simulink model "semi_GSTA"  (R2018b)
settings: Solver=FixedStepAuto  StartTime=0.0  StopTime=100  FixedStep=0.01  RelTol=1e-3
InitFcn:
  | parameters_semi_const_noise
model workspace: external: MAT-File (data not in the file)
undefined symbols (not defined in the file or in its folder): eta0, ev_sampling_time, fig_st, h_ATD, h_ATD_sds, Mn, st_controller, T0, v0, x1, x2, x3, x4, x5, x6
libraries: sdolib x6, simulink x1
(part 6 of 6)

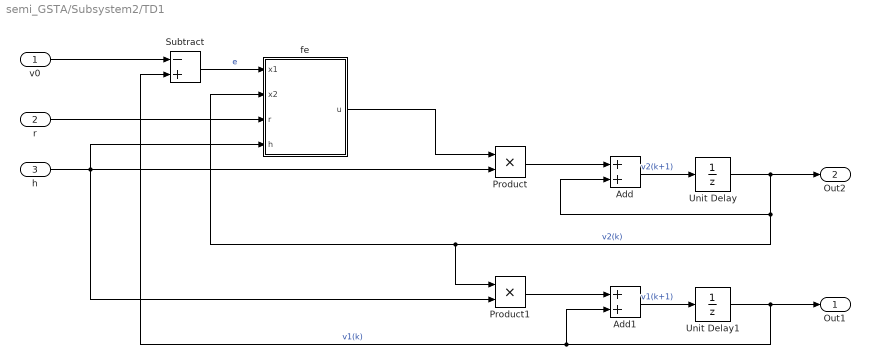
== system semi_GSTA/Subsystem2/TD1 ==
  v0 : Inport
  r : Inport  Port=2
  h : Inport  Port=3
  Add : Sum
  Add1 : Sum
  Product : Product  RndMeth=Zero
  Product1 : Product  RndMeth=Zero
  Subtract : Sum  Inputs=-+
  Unit Delay : UnitDelay  SampleTime=-1
  Unit Delay1 : UnitDelay  InitialCondition=eta0(1)  SampleTime=-1
  fe : MATLAB Function  TreatAsAtomicUnit=on
  Out1 : Outport
  Out2 : Outport  Port=2
  wires:
  v0/1 -> Subtract/1
  Subtract/1 -> fe/1(x1)  "e"
  r/1 -> fe/3(r)
  h/1 -> Product/2, fe/4(h), Product1/2
  fe/1(u) -> Product/1
  Product/1 -> Add/1
  Add/1 -> Unit Delay/1  "v2(k+1)"
  Unit Delay/1 -> Add/2, Product1/1, fe/2(x2), Out2/1  "v2(k)"
  Add1/1 -> Unit Delay1/1  "v1(k+1)"
  Unit Delay1/1 -> Out1/1, Add1/2, Subtract/2  "v1(k)"
  Product1/1 -> Add1/1

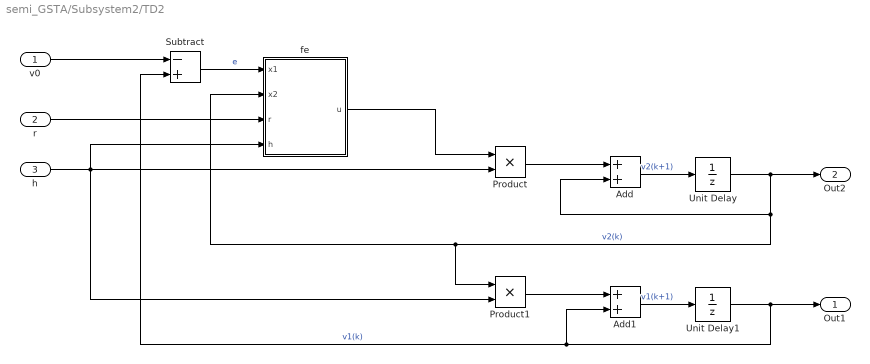
== system semi_GSTA/Subsystem2/TD2 ==
  v0 : Inport
  r : Inport  Port=2
  h : Inport  Port=3
  Add : Sum
  Add1 : Sum
  Product : Product  RndMeth=Zero
  Product1 : Product  RndMeth=Zero
  Subtract : Sum  Inputs=-+
  Unit Delay : UnitDelay  SampleTime=-1
  Unit Delay1 : UnitDelay  InitialCondition=eta0(2)  SampleTime=-1
  fe : MATLAB Function  TreatAsAtomicUnit=on
  Out1 : Outport
  Out2 : Outport  Port=2
  wires:
  Product1/1 -> Add1/1
  Unit Delay1/1 -> Subtract/2, Add1/2, Out1/1  "v1(k)"
  Add1/1 -> Unit Delay1/1  "v1(k+1)"
  Unit Delay/1 -> Out2/1, fe/2(x2), Product1/1, Add/2  "v2(k)"
  Add/1 -> Unit Delay/1  "v2(k+1)"
  Product/1 -> Add/1
  fe/1(u) -> Product/1
  h/1 -> Product1/2, fe/4(h), Product/2
  r/1 -> fe/3(r)
  Subtract/1 -> fe/1(x1)  "e"
  v0/1 -> Subtract/1

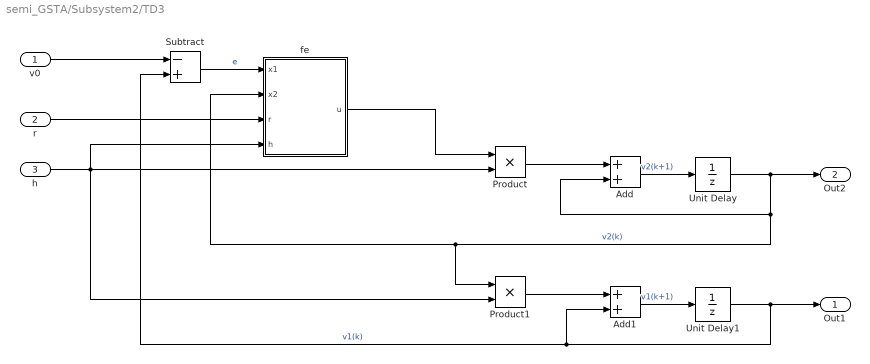
== system semi_GSTA/Subsystem2/TD3 ==
  v0 : Inport
  r : Inport  Port=2
  h : Inport  Port=3
  Add : Sum
  Add1 : Sum
  Product : Product  RndMeth=Zero
  Product1 : Product  RndMeth=Zero
  Subtract : Sum  Inputs=-+
  Unit Delay : UnitDelay  SampleTime=-1
  Unit Delay1 : UnitDelay  InitialCondition=eta0(3)  SampleTime=-1
  fe : MATLAB Function  TreatAsAtomicUnit=on
  Out1 : Outport
  Out2 : Outport  Port=2
  wires:
  v0/1 -> Subtract/1
  Subtract/1 -> fe/1(x1)  "e"
  r/1 -> fe/3(r)
  h/1 -> Product/2, fe/4(h), Product1/2
  fe/1(u) -> Product/1
  Product/1 -> Add/1
  Add/1 -> Unit Delay/1  "v2(k+1)"
  Unit Delay/1 -> Add/2, Product1/1, fe/2(x2), Out2/1  "v2(k)"
  Add1/1 -> Unit Delay1/1  "v1(k+1)"
  Unit Delay1/1 -> Out1/1, Add1/2, Subtract/2  "v1(k)"
  Product1/1 -> Add1/1

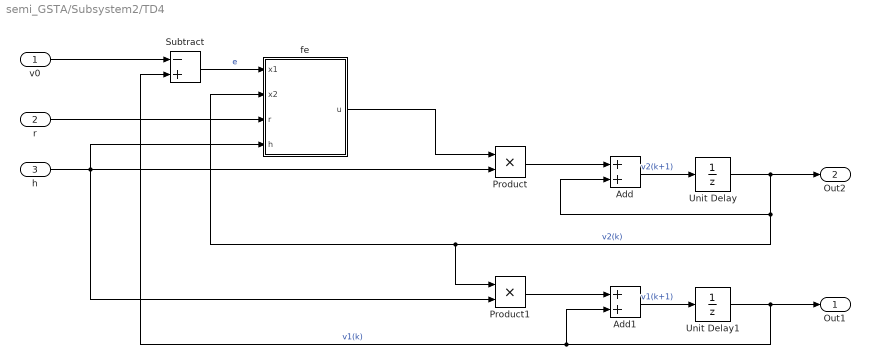
== system semi_GSTA/Subsystem2/TD4 ==
  v0 : Inport
  r : Inport  Port=2
  h : Inport  Port=3
  Add : Sum
  Add1 : Sum
  Product : Product  RndMeth=Zero
  Product1 : Product  RndMeth=Zero
  Subtract : Sum  Inputs=-+
  Unit Delay : UnitDelay  SampleTime=-1
  Unit Delay1 : UnitDelay  InitialCondition=eta0(4)  SampleTime=-1
  fe : MATLAB Function  TreatAsAtomicUnit=on
  Out1 : Outport
  Out2 : Outport  Port=2
  wires:
  Product1/1 -> Add1/1
  Unit Delay1/1 -> Subtract/2, Add1/2, Out1/1  "v1(k)"
  Add1/1 -> Unit Delay1/1  "v1(k+1)"
  Unit Delay/1 -> Out2/1, fe/2(x2), Product1/1, Add/2  "v2(k)"
  Add/1 -> Unit Delay/1  "v2(k+1)"
  Product/1 -> Add/1
  fe/1(u) -> Product/1
  h/1 -> Product1/2, fe/4(h), Product/2
  r/1 -> fe/3(r)
  Subtract/1 -> fe/1(x1)  "e"
  v0/1 -> Subtract/1

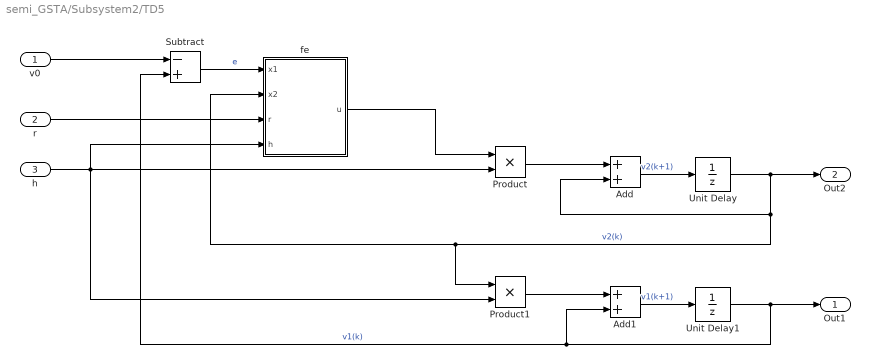
== system semi_GSTA/Subsystem2/TD5 ==
  v0 : Inport
  r : Inport  Port=2
  h : Inport  Port=3
  Add : Sum
  Add1 : Sum
  Product : Product  RndMeth=Zero
  Product1 : Product  RndMeth=Zero
  Subtract : Sum  Inputs=-+
  Unit Delay : UnitDelay  SampleTime=-1
  Unit Delay1 : UnitDelay  InitialCondition=eta0(5)  SampleTime=-1
  fe : MATLAB Function  TreatAsAtomicUnit=on
  Out1 : Outport
  Out2 : Outport  Port=2
  wires:
  v0/1 -> Subtract/1
  Subtract/1 -> fe/1(x1)  "e"
  r/1 -> fe/3(r)
  h/1 -> Product/2, fe/4(h), Product1/2
  fe/1(u) -> Product/1
  Product/1 -> Add/1
  Add/1 -> Unit Delay/1  "v2(k+1)"
  Unit Delay/1 -> Add/2, Product1/1, fe/2(x2), Out2/1  "v2(k)"
  Add1/1 -> Unit Delay1/1  "v1(k+1)"
  Unit Delay1/1 -> Out1/1, Add1/2, Subtract/2  "v1(k)"
  Product1/1 -> Add1/1

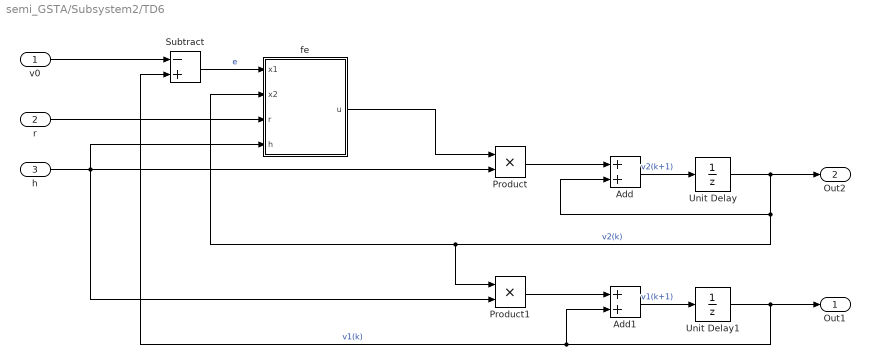
== system semi_GSTA/Subsystem2/TD6 ==
  v0 : Inport
  r : Inport  Port=2
  h : Inport  Port=3
  Add : Sum
  Add1 : Sum
  Product : Product  RndMeth=Zero
  Product1 : Product  RndMeth=Zero
  Subtract : Sum  Inputs=-+
  Unit Delay : UnitDelay  SampleTime=-1
  Unit Delay1 : UnitDelay  InitialCondition=eta0(6)  SampleTime=-1
  fe : MATLAB Function  TreatAsAtomicUnit=on
  Out1 : Outport
  Out2 : Outport  Port=2
  wires:
  Product1/1 -> Add1/1
  Unit Delay1/1 -> Subtract/2, Add1/2, Out1/1  "v1(k)"
  Add1/1 -> Unit Delay1/1  "v1(k+1)"
  Unit Delay/1 -> Out2/1, fe/2(x2), Product1/1, Add/2  "v2(k)"
  Add/1 -> Unit Delay/1  "v2(k+1)"
  Product/1 -> Add/1
  fe/1(u) -> Product/1
  h/1 -> Product1/2, fe/4(h), Product/2
  r/1 -> fe/3(r)
  Subtract/1 -> fe/1(x1)  "e"
  v0/1 -> Subtract/1

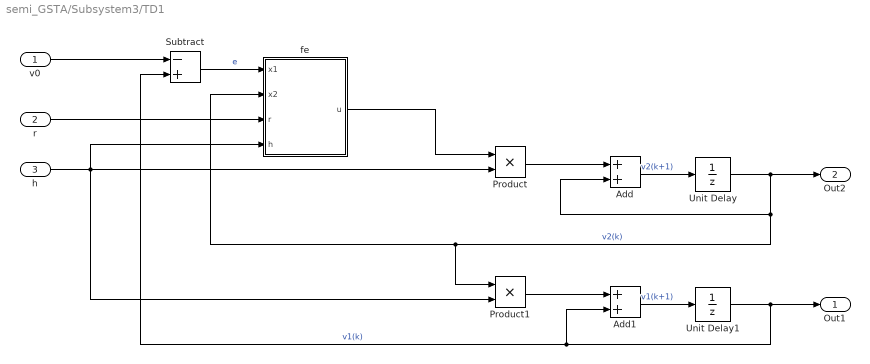
== system semi_GSTA/Subsystem3/TD1 ==
  v0 : Inport
  r : Inport  Port=2
  h : Inport  Port=3
  Add : Sum
  Add1 : Sum
  Product : Product  RndMeth=Zero
  Product1 : Product  RndMeth=Zero
  Subtract : Sum  Inputs=-+
  Unit Delay : UnitDelay  SampleTime=-1
  Unit Delay1 : UnitDelay  InitialCondition=eta0(1)  SampleTime=-1
  fe : MATLAB Function  TreatAsAtomicUnit=on
  Out1 : Outport
  Out2 : Outport  Port=2
  wires:
  Product1/1 -> Add1/1
  Unit Delay1/1 -> Subtract/2, Add1/2, Out1/1  "v1(k)"
  Add1/1 -> Unit Delay1/1  "v1(k+1)"
  Unit Delay/1 -> Out2/1, fe/2(x2), Product1/1, Add/2  "v2(k)"
  Add/1 -> Unit Delay/1  "v2(k+1)"
  Product/1 -> Add/1
  fe/1(u) -> Product/1
  h/1 -> Product1/2, fe/4(h), Product/2
  r/1 -> fe/3(r)
  Subtract/1 -> fe/1(x1)  "e"
  v0/1 -> Subtract/1

== system semi_GSTA/Subsystem3/TD2 ==
  v0 : Inport
  r : Inport  Port=2
  h : Inport  Port=3
  Add : Sum
  Add1 : Sum
  Product : Product  RndMeth=Zero
  Product1 : Product  RndMeth=Zero
  Subtract : Sum  Inputs=-+
  Unit Delay : UnitDelay  SampleTime=-1
  Unit Delay1 : UnitDelay  InitialCondition=eta0(2)  SampleTime=-1
  fe : MATLAB Function  TreatAsAtomicUnit=on
  Out1 : Outport
  Out2 : Outport  Port=2
  wires:
  v0/1 -> Subtract/1
  Subtract/1 -> fe/1(x1)  "e"
  r/1 -> fe/3(r)
  h/1 -> Product/2, fe/4(h), Product1/2
  fe/1(u) -> Product/1
  Product/1 -> Add/1
  Add/1 -> Unit Delay/1  "v2(k+1)"
  Unit Delay/1 -> Add/2, Product1/1, fe/2(x2), Out2/1  "v2(k)"
  Add1/1 -> Unit Delay1/1  "v1(k+1)"
  Unit Delay1/1 -> Out1/1, Add1/2, Subtract/2  "v1(k)"
  Product1/1 -> Add1/1

== system semi_GSTA/Subsystem3/TD3 ==
  v0 : Inport
  r : Inport  Port=2
  h : Inport  Port=3
  Add : Sum
  Add1 : Sum
  Product : Product  RndMeth=Zero
  Product1 : Product  RndMeth=Zero
  Subtract : Sum  Inputs=-+
  Unit Delay : UnitDelay  SampleTime=-1
  Unit Delay1 : UnitDelay  InitialCondition=eta0(3)  SampleTime=-1
  fe : MATLAB Function  TreatAsAtomicUnit=on
  Out1 : Outport
  Out2 : Outport  Port=2
  wires:
  Product1/1 -> Add1/1
  Unit Delay1/1 -> Subtract/2, Add1/2, Out1/1  "v1(k)"
  Add1/1 -> Unit Delay1/1  "v1(k+1)"
  Unit Delay/1 -> Out2/1, fe/2(x2), Product1/1, Add/2  "v2(k)"
  Add/1 -> Unit Delay/1  "v2(k+1)"
  Product/1 -> Add/1
  fe/1(u) -> Product/1
  h/1 -> Product1/2, fe/4(h), Product/2
  r/1 -> fe/3(r)
  Subtract/1 -> fe/1(x1)  "e"
  v0/1 -> Subtract/1

== system semi_GSTA/Subsystem3/TD4 ==
  v0 : Inport
  r : Inport  Port=2
  h : Inport  Port=3
  Add : Sum
  Add1 : Sum
  Product : Product  RndMeth=Zero
  Product1 : Product  RndMeth=Zero
  Subtract : Sum  Inputs=-+
  Unit Delay : UnitDelay  SampleTime=-1
  Unit Delay1 : UnitDelay  InitialCondition=eta0(4)  SampleTime=-1
  fe : MATLAB Function  TreatAsAtomicUnit=on
  Out1 : Outport
  Out2 : Outport  Port=2
  wires:
  v0/1 -> Subtract/1
  Subtract/1 -> fe/1(x1)  "e"
  r/1 -> fe/3(r)
  h/1 -> Product/2, fe/4(h), Product1/2
  fe/1(u) -> Product/1
  Product/1 -> Add/1
  Add/1 -> Unit Delay/1  "v2(k+1)"
  Unit Delay/1 -> Add/2, Product1/1, fe/2(x2), Out2/1  "v2(k)"
  Add1/1 -> Unit Delay1/1  "v1(k+1)"
  Unit Delay1/1 -> Out1/1, Add1/2, Subtract/2  "v1(k)"
  Product1/1 -> Add1/1

== system semi_GSTA/Subsystem3/TD5 ==
  v0 : Inport
  r : Inport  Port=2
  h : Inport  Port=3
  Add : Sum
  Add1 : Sum
  Product : Product  RndMeth=Zero
  Product1 : Product  RndMeth=Zero
  Subtract : Sum  Inputs=-+
  Unit Delay : UnitDelay  SampleTime=-1
  Unit Delay1 : UnitDelay  InitialCondition=eta0(5)  SampleTime=-1
  fe : MATLAB Function  TreatAsAtomicUnit=on
  Out1 : Outport
  Out2 : Outport  Port=2
  wires:
  Product1/1 -> Add1/1
  Unit Delay1/1 -> Subtract/2, Add1/2, Out1/1  "v1(k)"
  Add1/1 -> Unit Delay1/1  "v1(k+1)"
  Unit Delay/1 -> Out2/1, fe/2(x2), Product1/1, Add/2  "v2(k)"
  Add/1 -> Unit Delay/1  "v2(k+1)"
  Product/1 -> Add/1
  fe/1(u) -> Product/1
  h/1 -> Product1/2, fe/4(h), Product/2
  r/1 -> fe/3(r)
  Subtract/1 -> fe/1(x1)  "e"
  v0/1 -> Subtract/1

== system semi_GSTA/Subsystem3/TD6 ==
  v0 : Inport
  r : Inport  Port=2
  h : Inport  Port=3
  Add : Sum
  Add1 : Sum
  Product : Product  RndMeth=Zero
  Product1 : Product  RndMeth=Zero
  Subtract : Sum  Inputs=-+
  Unit Delay : UnitDelay  SampleTime=-1
  Unit Delay1 : UnitDelay  InitialCondition=eta0(6)  SampleTime=-1
  fe : MATLAB Function  TreatAsAtomicUnit=on
  Out1 : Outport
  Out2 : Outport  Port=2
  wires:
  v0/1 -> Subtract/1
  Subtract/1 -> fe/1(x1)  "e"
  r/1 -> fe/3(r)
  h/1 -> Product/2, fe/4(h), Product1/2
  fe/1(u) -> Product/1
  Product/1 -> Add/1
  Add/1 -> Unit Delay/1  "v2(k+1)"
  Unit Delay/1 -> Add/2, Product1/1, fe/2(x2), Out2/1  "v2(k)"
  Add1/1 -> Unit Delay1/1  "v1(k+1)"
  Unit Delay1/1 -> Out1/1, Add1/2, Subtract/2  "v1(k)"
  Product1/1 -> Add1/1

== matlab function semi_GSTA/MATLAB Function2 ==
  data: vx input; eta input; deta input; ddeta input; fx output; mdis_c input; edis input; Mn input
function fx= total_disturbance(vx,eta,deta,ddeta, mdis_c,edis,Mn)

ux=vx(1); v=vx(2); w=vx(3); p=vx(4); q=vx(5); r=vx(6);

fa=eta(4); th=eta(5); psi=eta(6);

dfa=deta(4); dth=deta(5); dpsi=deta(6);

%基本参数
ds=pi/2;

cg=0.001*[-16.9331   -1.7786   -3.3727];
cb=0.001*[-6.8888   -0.8305   -1.5036];

xG=cg(1); yG=cg(2); zG=cg(3);  
xB=cb(1);  yB=cb(2);  zB=cb(3);

g=9.8; rou=1027.77;
m=4.2631e+03;   W=m*g;    B=4.3007e+03*g;
Ix=999; Iy=4036; Iz=3703; Ixy=0; Iyz=0; Ixz=38;
%

%%水动力系数
Xu=-0.601400991132054*rou;  Xv=0.114602622907669*rou;  Xw=0.0313912897542816*rou; Xq=-0.345363159830523*rou; Xr=0.00797347338964364*rou; Xds=1.14776823525357*rou; 
Xdu=-1.41861604806325*rou; Xdv=0.0509196259090768*rou; Xdw=0.062564375040305*rou; Xdq=0.16459042409977*rou; Xdr=0.072701596631006*rou;
Xvv=-2.56422118073801*rou;  Xuw=-0.193834998316606*rou; 

Yu=0.044394692600938*rou; Yv=-4.19928019864105*rou; Yr=0.753050700153444*rou; 
Ydu=-0.116693274950696*rou; Ydv=-12.0055397094293*rou; Ydr=1.36139005524804*rou; 
Yvv=7.25667282405077*rou; 

Zu=-0.352307725748354*rou; Zw=-0.61745690594626*rou; Zq=0.231237327207963*rou;
Zdu=-0.0292595216923672*rou; Zdw=-3.08486834519152*rou;  Zdq=-1.17435824946087*rou; 
Zww=-0.343307176159024*rou; Zdsds=-0.966615794554648*rou; 

Kv=-0.307241726736607*rou;  Kw=-0.11410490681724*rou;  Kp=-0.179037809260359*rou; 
Kdv=0.0483243873668225*rou; Kdw=0.0300470712066895*rou; Kdp=-0.347129493020368*rou; 
Kuw=-0.270819919475162*rou; 

Mu=0.00601107427170571*rou; Mw=0.000213173005733108*rou; Mq=-0.773559659457138*rou;  Mds=-0.0504865931950048*rou;
Mdu=-0.0608694810563339*rou; Mdw=0.427751472101112*rou; Mdq=-1.93011015874768*rou; 
Muw=1.27118217014846*rou; Mww=-0.149654360933358*rou; Mdsds=-1.77512548973347*rou; 

Nu=0.00618430827275825*rou; Nv=1.31787983106965*rou; Nr=-2.12059813452114*rou;
Ndu=0.00432067452610559*rou; Ndv=2.54908610448936*rou; Ndr=-5.08662579871407*rou; 
Nvv=-0.599395502737668*rou;

 %刚体的质量惯性矩阵MRB
MRB=[m 0 0 0 m*zG -m*yG
     0 m 0 -m*zG 0 m*xG
     0 0 m m*yG -m*xG 0
     0 -m*zG m*yG Ix -Ixy -Ixz
     m*zG 0 -m*xG -Ixy Iy -Iyz
     -m*yG m*xG 0 -Ixz -Iyz Iz];   
%附加质量惯性矩阵
MA=-[Xdu Xdv Xdw 0 Xdq Xdr
           Ydu Ydv  0 0 0 Ydr
           Zdu 0 Zdw 0 Zdq 0
           0 Kdv Kdw Kdp 0 0
           Mdu 0 Mdw 0 Mdq 0
           Ndu Ndv 0 0 0 Ndr];        
Mv=MRB+MA;       

 %科里奥利力和向心力矩阵CRBv=Cv
 Cv=[0 0 0 m*(yG*q+zG*r) m*(w-xG*q) -m*(xG*r+v)
         0 0 0 -m*(w+yG*p) m*(zG*r+xG*p) m*(ux-yG*r)
         0 0 0 m*(v-zG*p) -m*(ux+zG*q) m*(xG*p+yG*q)
        -m*(yG*q+zG*r) m*(w+yG*p) m*(zG*p-v) 0 -Iyz*q-Ixz*p+Iz*r Iyz*r+Ixy*p-Iy*q
          m*(xG*q-w) -m*(zG*r+xG*p) m*(ux+zG*q) Iyz*q+Ixz*p-Iz*r 0 -Ixz*r-Ixy*q+Ix*p
          m*(xG*r+v) m*(yG*r-ux) -m*(xG*p+yG*q) -Iyz*r-Ixy*p+Iy*q Ixz*r+Ixy*q-Ix*p 0];
      
%粘滞阻力
Dv=-[Xu+Xuw*abs(w), Xv+Xvv*abs(v), Xw+Xds*(ds-pi/2*sign(ds))*abs(w), 0, Xq, Xr;
         Yu, Yv+Yvv*abs(v), 0, 0, 0, Yr;
         Zu, 0, Zw+Zww*abs(w)+Zdsds*(ds-pi/2*sign(ds))^2*abs(w), 0, Zq, 0;
         Kuw*abs(w), Kv, Kw, Kp, 0, 0;
         Mu+Muw*w, 0, Mw+Mww*abs(w)+Mdsds*(ds-pi/2*sign(ds))^2*abs(w)+Mds*(ds-pi/2*sign(ds))*w, 0, Mq, 0;
         Nu, Nv+Nvv*abs(v), 0, 0, 0, Nr];

%载体的恢复力/力矩
gv=[(W-B)*sin(th)
    -(W-B)*cos(th)*sin(fa)
    -(W-B)*cos(th)*cos(fa) 
    -(yG*W-yB*B)*cos(th)*cos(fa)+(zG*W-zB*B)*cos(th)*sin(fa)
    (zG*W-zB*B)*sin(th)+(xG*W-xB*B)*cos(th)*cos(fa)
    -(xG*W-xB*B)*cos(th)*sin(fa)-(yG*W-yB*B)*sin(th)];

%雅可比矩阵

JT=[cos(psi)*cos(th),sin(psi)*cos(th),-sin(th),0,0,0;
          cos(psi)*sin(th)*sin(fa)-sin(psi)*cos(fa), cos(psi)*cos(fa)+sin(fa)*sin(th)*sin(psi),cos(th)*sin(fa),0,0,0;
          sin(psi)*sin(fa)+cos(psi)*cos(fa)*sin(th), sin(th)*sin(psi)*cos(fa)-cos(psi)*sin(fa),cos(th)*cos(fa),0,0,0;
          0,0,0,1,0,0;
          0,0,0,sin(fa)*tan(th),cos(fa),sin(fa)/cos(th);
          0,0,0,cos(fa)*tan(th), -sin(fa),cos(fa)/cos(th)]; 
invJ=[cos(psi)*cos(th),sin(psi)*cos(th),-sin(th),0,0,0;
          cos(psi)*sin(th)*sin(fa)-sin(psi)*cos(fa), cos(psi)*cos(fa)+sin(fa)*sin(th)*sin(psi),cos(th)*sin(fa),0,0,0;
          sin(psi)*sin(fa)+cos(psi)*cos(fa)*sin(th), sin(th)*sin(psi)*cos(fa)-cos(psi)*sin(fa),cos(th)*cos(fa),0,0,0;
          0,0,0,1,0,-sin(th);
          0,0,0,0,cos(fa),sin(fa)*cos(th);
          0,0,0,0,-sin(fa),cos(fa)*cos(th)]; 
invJT=[cos(psi)*cos(th), cos(psi)*sin(th)*sin(fa)-sin(psi)*cos(fa), sin(psi)*sin(fa)+cos(psi)*cos(fa)*sin(th),0,0,0;
            sin(psi)*cos(th), cos(psi)*cos(fa)+sin(fa)*sin(th)*sin(psi),sin(th)*sin(psi)*cos(fa)-cos(psi)*sin(fa),0,0,0;
           -sin(th), cos(th)*sin(fa), cos(th)*cos(fa),0,0,0;
           0,0,0,1,0,0;
           0,0,0,0,cos(fa),-sin(fa);
           0,0,0,-sin(th),sin(fa)*cos(th),cos(fa)*cos(th)]; 
       
 %雅可比矩阵的导数，不清楚正不正确

dJ1=[0,sin(psi)*sin(fa)+cos(psi)*sin(th)*cos(fa),sin(psi)*cos(fa)-cos(psi)*sin(fa)*sin(th),0,0,0;
         0,-cos(psi)*sin(fa)+cos(fa)*sin(th)*sin(psi),-cos(psi)*cos(fa)-sin(th)*sin(psi)*sin(fa),0,0,0;
         0,cos(th)*cos(fa),-cos(th)*sin(fa),0,0,0;
         0,0,0,0,cos(fa)*tan(th),-sin(fa)*tan(th);
         0,0,0,0,-sin(fa),-cos(fa);
         0,0,0,0,cos(fa)/cos(th),-sin(fa)/cos(th)];  

dJ2=[-cos(psi)*sin(th),cos(psi)*cos(th)*sin(fa),cos(psi)*cos(fa)*cos(th),0,0,0;
          -sin(psi)*sin(th),sin(fa)*cos(th)*sin(psi),cos(th)*sin(psi)*cos(fa),0,0,0;
          -cos(th),-sin(th)*sin(fa),-sin(th)*cos(fa),0,0,0;
            0,0,0,0,sin(fa)*sec(th)^2,cos(fa)*sec(th)^2;
            0,0,0,0,0,0;
            0,0,0,0,sin(fa)*sec(th)*tan(th),cos(fa)*sec(th)*tan(th) ];

dJ3=[-sin(psi)*cos(th),-cos(psi)*cos(fa)-sin(psi)*sin(th)*sin(fa),cos(psi)*sin(fa)-sin(psi)*cos(fa)*sin(th),0,0,0;
          cos(psi)*cos(th),-sin(psi)*cos(fa)+sin(fa)*sin(th)*cos(psi),sin(psi)*sin(fa)+sin(th)*cos(psi)*cos(fa),0,0,0;    
          0,0,0,0,0,0;
          0,0,0,0,0,0;
          0,0,0,0,0,0;
          0,0,0,0,0,0];
dJ=dfa*dJ1+dth*dJ2+dpsi*dJ3;  

%名义值：运动坐标系转换到惯性坐标系下
% M=(1-0.4)*invJT*Mv*invJ;
% C=(1+0.4)*invJT*(Cv-Mv*invJ*dJ)*invJ;
% D=(1-0.4)*invJT*Dv*invJ;
% g=(1-0.2)*invJT*gv;
% mdisn=0.6*invJT*mdis_c;

M=invJT*Mv*invJ;
% Mn=0.8*invJT*Mv*invJ;

C=invJT*(Cv-Mv*invJ*dJ)*invJ;
D=invJT*Dv*invJ;
g=invJT*gv;
mdisn=invJT*mdis_c;
edisn=invJT*edis;

%估算的S值
% fx=-inv(Mn)*(C*deta+D*deta+g-mdisn-edisn)-inv(Mn)*(M-Mn)*ddeta;
fx=-(C*deta+D*deta+g-mdisn-edisn)-(M-Mn)*ddeta;
end

== matlab function semi_GSTA/MATLAB Function4 ==
  data: detad input; deta input; ddeta input; ddetad input; ds output; c input
function ds = sliding_face(detad,deta,ddeta,ddetad,c)

ddeta=0;

de=deta-detad;
dde=ddeta-ddetad;
C=diag(c);

ds=dde+C*de;

== matlab function semi_GSTA/MATLAB Function5 ==
  data: etad input; eta input; s output; deta input; detad input; c input
function s= sliding_face(etad,eta,deta,detad,c)


e=eta-etad;
de=deta-detad;
C=diag(c);

s=de+C*e;

== matlab function semi_GSTA/ARV Dynamic Model3/MATLAB Function ==
  data: Tv input; mdis input; edis input; vx input; dv output; eta input; deta output
function [dv,deta] = Dynamics_vehicle(Tv, mdis, edis, vx, eta)

ux =vx(1); v = vx(2); w = vx(3); p = vx(4); q = vx(5); r = vx(6);

fa = eta(4); th= eta(5); psi = eta(6);

ds=pi/2;

cg=0.001*[-16.9331   -1.7786   -3.3727];
cb=0.001*[-6.8888   -0.8305   -1.5036];


xG=cg(1); yG=cg(2); zG=cg(3);  
xB=cb(1);  yB=cb(2);  zB=cb(3);

g=9.8; rou=1027.77;
m=4.2631e+03;   W=m*g;    B=4.3007e+03*g;
Ix=999; Iy=4036; Iz=3703; Ixy=0; Iyz=0; Ixz=38;

% hydrodynamic derivatives
Xu=-0.601400991132054*rou;  Xv=0.114602622907669*rou;  Xw=0.0313912897542816*rou; Xq=-0.345363159830523*rou; Xr=0.00797347338964364*rou; 
Xdu=-1.41861604806325*rou; Xdv=0.0509196259090768*rou; Xdw=0.062564375040305*rou; Xdq=0.16459042409977*rou; Xdr=0.072701596631006*rou;
Xvv=-2.56422118073801*rou;  Xuw=-0.193834998316606*rou; Xds=1.14776823525357*rou; 

Yu=0.044394692600938*rou; Yv=-4.19928019864105*rou; Yr=0.753050700153444*rou; 
Ydu=-0.116693274950696*rou; Ydv=-12.0055397094293*rou; Ydr=1.36139005524804*rou; 
Yvv=7.25667282405077*rou; 

Zu=-0.352307725748354*rou; Zw=-0.61745690594626*rou; Zq=0.231237327207963*rou;
Zdu=-0.0292595216923672*rou; Zdw=-3.08486834519152*rou;  Zdq=-1.17435824946087*rou; 
Zww=-0.343307176159024*rou; Zdsds=-0.966615794554648*rou; 

Kv=-0.307241726736607*rou;  Kw=-0.11410490681724*rou;  Kp=-0.179037809260359*rou; 
Kdv=0.0483243873668225*rou; Kdw=0.0300470712066895*rou; Kdp=-0.347129493020368*rou; 
Kuw=-0.270819919475162*rou; 

Mu=0.00601107427170571*rou; Mw=0.000213173005733108*rou; Mq=-0.773559659457138*rou;  
Mdu=-0.0608694810563339*rou; Mdw=0.427751472101112*rou; Mdq=-1.93011015874768*rou; 
Muw=1.27118217014846*rou; Mww=-0.149654360933358*rou; Mdsds=-1.77512548973347*rou; Mds=-0.0504865931950048*rou;

Nu=0.00618430827275825*rou; Nv=1.31787983106965*rou; Nr=-2.12059813452114*rou;
Ndu=0.00432067452610559*rou; Ndv=2.54908610448936*rou; Ndr=-5.08662579871407*rou; 
Nvv=-0.599395502737668*rou;


% model parameter matrix
J=[cos(psi)*cos(th), cos(psi)*sin(th)*sin(fa)-sin(psi)*cos(fa), sin(psi)*sin(fa)+cos(psi)*cos(fa)*sin(th),0,0,0;
   sin(psi)*cos(th), cos(psi)*cos(fa)+sin(fa)*sin(th)*sin(psi),sin(th)*sin(psi)*cos(fa)-cos(psi)*sin(fa),0,0,0;
   -sin(th), cos(th)*sin(fa), cos(th)*cos(fa),0,0,0;
   0,0,0,1,sin(fa)*tan(th),cos(fa)*tan(th);
   0,0,0,0,cos(fa),-sin(fa);
   0,0,0,0,sin(fa)*sec(th),cos(fa)*sec(th)];  

        
%刚体的质量惯性矩阵MRB
MRB=[m 0 0 0 m*zG -m*yG
     0 m 0 -m*zG 0 m*xG
     0 0 m m*yG -m*xG 0
     0 -m*zG m*yG Ix -Ixy -Ixz
     m*zG 0 -m*xG -Ixy Iy -Iyz
     -m*yG m*xG 0 -Ixz -Iyz Iz];
 %科里奥利力和向心力矩阵CRBv=Cv
 Cv= [0 0 0 m*(yG*q+zG*r) m*(w-xG*q) -m*(xG*r+v)
         0 0 0 -m*(w+yG*p) m*(zG*r+xG*p) m*(ux-yG*r)
         0 0 0 m*(v-zG*p) -m*(ux+zG*q) m*(xG*p+yG*q)
        -m*(yG*q+zG*r) m*(w+yG*p) m*(zG*p-v) 0 -Iyz*q-Ixz*p+Iz*r Iyz*r+Ixy*p-Iy*q
          m*(xG*q-w) -m*(zG*r+xG*p) m*(ux+zG*q) Iyz*q+Ixz*p-Iz*r 0 -Ixz*r-Ixy*q+Ix*p
          m*(xG*r+v) m*(yG*r-ux) -m*(xG*p+yG*q) -Iyz*r-Ixy*p+Iy*q Ixz*r+Ixy*q-Ix*p 0];
      
%附加质量惯性矩阵
MA=-[Xdu Xdv Xdw 0 Xdq Xdr
           Ydu Ydv  0 0 0 Ydr
           Zdu 0 Zdw 0 Zdq 0
           0 Kdv Kdw Kdp 0 0
           Mdu 0 Mdw 0 Mdq 0
           Ndu Ndv 0 0 0 Ndr]; 
       
Mv=MRB+MA;

%粘滞阻力
Dv=-[Xu+Xuw*abs(w), Xv+Xvv*abs(v), Xw+Xds*(ds-pi/2*sign(ds))*abs(w), 0, Xq, Xr;
         Yu, Yv+Yvv*abs(v), 0, 0, 0, Yr;
         Zu, 0, Zw+Zww*abs(w)+Zdsds*(ds-pi/2*sign(ds))^2*abs(w), 0, Zq, 0;
         Kuw*abs(w), Kv, Kw, Kp, 0, 0;
         Mu+Muw*w, 0, Mw+Mww*abs(w)+Mdsds*(ds-pi/2*sign(ds))^2*abs(w)+Mds*(ds-pi/2*sign(ds))*w, 0, Mq, 0;
         Nu, Nv+Nvv*abs(v), 0, 0, 0, Nr];

%载体的恢复力/力矩
gv=[(W-B)*sin(th)
      -(W-B)*cos(th)*sin(fa)
      -(W-B)*cos(th)*cos(fa) 
      -(yG*W-yB*B)*cos(th)*cos(fa)+(zG*W-zB*B)*cos(th)*sin(fa)
       (zG*W-zB*B)*sin(th)+(xG*W-xB*B)*cos(th)*cos(fa)
      -(xG*W-xB*B)*cos(th)*sin(fa)-(yG*W-yB*B)*sin(th)];


dv=Mv\(Tv+mdis+edis-Cv*vx-Dv*vx-gv);
deta=J*vx;

== matlab function semi_GSTA/Subsystem3/TD1/fe ==
  data: x1 input; u output; x2 input; r input; h input
function u=fhan(x1,x2,r,h)
%eml
d=r*h*h;
a0=h*x2;
y=x1+a0;
a1=(d*(d+8*abs(y)))^0.5;
a2=a0+sign(y)*(a1-d)*0.5;
a=(a0+y)*(sign(y+d)-sign(y-d))*0.5+a2*(1-(sign(y+d)-sign(y-d))*0.5);
u=-r*(a/d)*(sign(a+d)-sign(a-d))*0.5-r*sign(a)*(1-(sign(a+d)-sign(a-d))*0.5);

== matlab function semi_GSTA/Adaptive law1/MATLAB Function2 ==
  data: v input; k1 input; s input; usta output; mu1 input; mu2 input
function usta= usta(v,k1,s,mu1,mu2)

usta=zeros(6,1);

for i=1:6
   usta(i)=-k1(i)*( mu1(i)*abs(s(i))^0.5*sign(s(i))+mu2(i)*s(i) )+v(i);
end




% d=0.01;
% sat=zeros(6,1);
% for i=1:6
%     if s(i)>d
%         sat(i)=1;
%     elseif s(i)<-d
%         sat(i)=-1;
%     else
%         sat(i)=s(i)/d;
%     end
%     
%    usta(i)=-k1(i)*( mu1(i)*abs(s(i))^0.5*sat(i)+mu2(i)*s(i) )+lam(i);
% end

== matlab function semi_GSTA/Adaptive law1/MATLAB Function4 ==
  data: h input; s input; k1_kp1 output; w input; delta input; k0 input; k1_k input
function k1_kp1= dk1(h,s,w,delta,k0, k1_k)

k1_kp1=zeros(6,1);


% % % % % % % % % % % % % % % % % % 


for i=1:6
 
if k1_k(i)==0
    k1_kp1(i)=k0(i);
elseif abs(s(i))<=delta(i)
    k1_kp1(i)=k1_k(i);   
else
    k1_kp1(i)=k1_k(i)+h*w(i);
end

end


% % % % % % % % % % % % % % % %

== matlab function semi_GSTA/Subsystem2/TD1/fe ==
  data: x1 input; u output; x2 input; r input; h input
function u=fhan(x1,x2,r,h)
%eml
d=r*h*h;
a0=h*x2;
y=x1+a0;
a1=(d*(d+8*abs(y)))^0.5;
a2=a0+sign(y)*(a1-d)*0.5;
a=(a0+y)*(sign(y+d)-sign(y-d))*0.5+a2*(1-(sign(y+d)-sign(y-d))*0.5);
u=-r*(a/d)*(sign(a+d)-sign(a-d))*0.5-r*sign(a)*(1-(sign(a+d)-sign(a-d))*0.5);

== matlab function semi_GSTA/MATLAB Function6 ==
  data: Tv input; tou output
function tou = thrust_allocation(Tv)

%理想化的全驱动，利用到了前面的侧推，不同的旋转推进器角度: 角度不同即可
x_stn=-1.722; y_stn=0.6; z_stn=-0.02;
x_bow=0.75;  y_bow=0.55231;  x_hB=0.8; x_hS=-1 ;

dsL=-72*pi/180; dsR=-55*pi/180;

B=[cos(dsL) cos(dsR)  0 0 0 0;
      0 0  1 1 0 0;
     -sin(dsL) -sin(dsR)  0 0 1 1;
     y_stn*sin(dsL)  -y_stn*sin(dsR)  0 0 -y_bow y_bow;
     z_stn*cos(dsL)+x_stn*sin(dsL)   z_stn*cos(dsR)+x_stn*sin(dsR)  0 0 -x_bow  -x_bow;
     y_stn*cos(dsL)  -y_stn*cos(dsR) x_hB x_hS 0 0];
 
% FsL,FsR,FhB,FhS,FbL,FbR
tou=B\Tv; 
% -1.00308844074030,-0.588501345539596   -57.4727  -33.7186

end

== matlab function semi_GSTA/MATLAB Function10 ==
  data: Tn input; Tv output; eta input
function Tv = Trans(Tn,eta)

fa=eta(4); th=eta(5); psi=eta(6);


JT=[cos(psi)*cos(th),sin(psi)*cos(th),-sin(th),0,0,0;
          cos(psi)*sin(th)*sin(fa)-sin(psi)*cos(fa), cos(psi)*cos(fa)+sin(fa)*sin(th)*sin(psi),cos(th)*sin(fa),0,0,0;
          sin(psi)*sin(fa)+cos(psi)*cos(fa)*sin(th), sin(th)*sin(psi)*cos(fa)-cos(psi)*sin(fa),cos(th)*cos(fa),0,0,0;
          0,0,0,1,0,0;
          0,0,0,sin(fa)*tan(th),cos(fa),sin(fa)/cos(th);
          0,0,0,cos(fa)*tan(th), -sin(fa),cos(fa)/cos(th)]; 

Tv=JT*Tn;


end

== matlab function semi_GSTA/Subsystem2/TD2/fe ==
  data: x1 input; u output; x2 input; r input; h input
function u=fhan(x1,x2,r,h)
%eml
d=r*h*h;
a0=h*x2;
y=x1+a0;
a1=(d*(d+8*abs(y)))^0.5;
a2=a0+sign(y)*(a1-d)*0.5;
a=(a0+y)*(sign(y+d)-sign(y-d))*0.5+a2*(1-(sign(y+d)-sign(y-d))*0.5);
u=-r*(a/d)*(sign(a+d)-sign(a-d))*0.5-r*sign(a)*(1-(sign(a+d)-sign(a-d))*0.5);

== matlab function semi_GSTA/Subsystem3/TD2/fe ==
  data: x1 input; u output; x2 input; r input; h input
function u=fhan(x1,x2,r,h)
%eml
d=r*h*h;
a0=h*x2;
y=x1+a0;
a1=(d*(d+8*abs(y)))^0.5;
a2=a0+sign(y)*(a1-d)*0.5;
a=(a0+y)*(sign(y+d)-sign(y-d))*0.5+a2*(1-(sign(y+d)-sign(y-d))*0.5);
u=-r*(a/d)*(sign(a+d)-sign(a-d))*0.5-r*sign(a)*(1-(sign(a+d)-sign(a-d))*0.5);

== matlab function semi_GSTA/Subsystem2/TD3/fe ==
  data: x1 input; u output; x2 input; r input; h input
function u=fhan(x1,x2,r,h)
%eml
d=r*h*h;
a0=h*x2;
y=x1+a0;
a1=(d*(d+8*abs(y)))^0.5;
a2=a0+sign(y)*(a1-d)*0.5;
a=(a0+y)*(sign(y+d)-sign(y-d))*0.5+a2*(1-(sign(y+d)-sign(y-d))*0.5);
u=-r*(a/d)*(sign(a+d)-sign(a-d))*0.5-r*sign(a)*(1-(sign(a+d)-sign(a-d))*0.5);

== matlab function semi_GSTA/Subsystem2/TD4/fe ==
  data: x1 input; u output; x2 input; r input; h input
function u=fhan(x1,x2,r,h)
%eml
d=r*h*h;
a0=h*x2;
y=x1+a0;
a1=(d*(d+8*abs(y)))^0.5;
a2=a0+sign(y)*(a1-d)*0.5;
a=(a0+y)*(sign(y+d)-sign(y-d))*0.5+a2*(1-(sign(y+d)-sign(y-d))*0.5);
u=-r*(a/d)*(sign(a+d)-sign(a-d))*0.5-r*sign(a)*(1-(sign(a+d)-sign(a-d))*0.5);

== matlab function semi_GSTA/Subsystem3/TD3/fe ==
  data: x1 input; u output; x2 input; r input; h input
function u=fhan(x1,x2,r,h)
%eml
d=r*h*h;
a0=h*x2;
y=x1+a0;
a1=(d*(d+8*abs(y)))^0.5;
a2=a0+sign(y)*(a1-d)*0.5;
a=(a0+y)*(sign(y+d)-sign(y-d))*0.5+a2*(1-(sign(y+d)-sign(y-d))*0.5);
u=-r*(a/d)*(sign(a+d)-sign(a-d))*0.5-r*sign(a)*(1-(sign(a+d)-sign(a-d))*0.5);

== matlab function semi_GSTA/Subsystem2/TD5/fe ==
  data: x1 input; u output; x2 input; r input; h input
function u=fhan(x1,x2,r,h)
%eml
d=r*h*h;
a0=h*x2;
y=x1+a0;
a1=(d*(d+8*abs(y)))^0.5;
a2=a0+sign(y)*(a1-d)*0.5;
a=(a0+y)*(sign(y+d)-sign(y-d))*0.5+a2*(1-(sign(y+d)-sign(y-d))*0.5);
u=-r*(a/d)*(sign(a+d)-sign(a-d))*0.5-r*sign(a)*(1-(sign(a+d)-sign(a-d))*0.5);

== matlab function semi_GSTA/Adaptive law1/MATLAB Function5 ==
  data: h input; mu1 input; mu2 input; eps input; beta input; s input; k2 output; k1 input; v_kp1 output; v_k input
function [k2,v_kp1]= dlam(h,mu1,mu2,eps,beta,s,k1,v_k)
k2=zeros(6,1);
fa2=zeros(6,1);
v_kp1=zeros(6,1);

for i=1:6
   fa2(i)=0.5*mu1(i)^2*sign(s(i))+1.5*mu1(i)*mu2(i)*abs(s(i))^0.5*sign(s(i))+mu2(i)^2*s(i);
   k2(i)=2*eps(i)*k1(i)+beta(i)+4*eps(i)^2;
   v_kp1(i)=v_k(i)-h*k2(i)*fa2(i);
end

== matlab function semi_GSTA/Subsystem2/TD6/fe ==
  data: x1 input; u output; x2 input; r input; h input
function u=fhan(x1,x2,r,h)
%eml
d=r*h*h;
a0=h*x2;
y=x1+a0;
a1=(d*(d+8*abs(y)))^0.5;
a2=a0+sign(y)*(a1-d)*0.5;
a=(a0+y)*(sign(y+d)-sign(y-d))*0.5+a2*(1-(sign(y+d)-sign(y-d))*0.5);
u=-r*(a/d)*(sign(a+d)-sign(a-d))*0.5-r*sign(a)*(1-(sign(a+d)-sign(a-d))*0.5);

== matlab function semi_GSTA/MATLAB Function3 ==
  data: vx input; eta input; deta input; fx output; mdis_c input
function fx= Model_nominal(vx,eta,deta,mdis_c)

ux=vx(1); v=vx(2); w=vx(3); p=vx(4); q=vx(5); r=vx(6);

fa=eta(4); th=eta(5); psi=eta(6);

dfa=deta(4); dth=deta(5); dpsi=deta(6);

ds=pi/2;

cg=0.001*[-16.9331   -1.7786   -3.3727];
cb=0.001*[-6.8888   -0.8305   -1.5036];


xG=cg(1); yG=cg(2); zG=cg(3);  
xB=cb(1);  yB=cb(2);  zB=cb(3);

g=9.8; rou=1027.77;
m=4.2631e+03;   W=m*g;    B=4.3007e+03*g;
Ix=999; Iy=4036; Iz=3703; Ixy=0; Iyz=0; Ixz=38;

%%水动力系数
Xu=-0.601400991132054*rou;  Xv=0.114602622907669*rou;  Xw=0.0313912897542816*rou; Xq=-0.345363159830523*rou; Xr=0.00797347338964364*rou; Xds=1.14776823525357*rou; 
Xdu=-1.41861604806325*rou; Xdv=0.0509196259090768*rou; Xdw=0.062564375040305*rou; Xdq=0.16459042409977*rou; Xdr=0.072701596631006*rou;
Xvv=-2.56422118073801*rou;  Xuw=-0.193834998316606*rou; 

Yu=0.044394692600938*rou; Yv=-4.19928019864105*rou; Yr=0.753050700153444*rou; 
Ydu=-0.116693274950696*rou; Ydv=-12.0055397094293*rou; Ydr=1.36139005524804*rou; 
Yvv=7.25667282405077*rou; 

Zu=-0.352307725748354*rou; Zw=-0.61745690594626*rou; Zq=0.231237327207963*rou;
Zdu=-0.0292595216923672*rou; Zdw=-3.08486834519152*rou;  Zdq=-1.17435824946087*rou; 
Zww=-0.343307176159024*rou; Zdsds=-0.966615794554648*rou; 

Kv=-0.307241726736607*rou;  Kw=-0.11410490681724*rou;  Kp=-0.179037809260359*rou; 
Kdv=0.0483243873668225*rou; Kdw=0.0300470712066895*rou; Kdp=-0.347129493020368*rou; 
Kuw=-0.270819919475162*rou; 

Mu=0.00601107427170571*rou; Mw=0.000213173005733108*rou; Mq=-0.773559659457138*rou;  Mds=-0.0504865931950048*rou;
Mdu=-0.0608694810563339*rou; Mdw=0.427751472101112*rou; Mdq=-1.93011015874768*rou; 
Muw=1.27118217014846*rou; Mww=-0.149654360933358*rou; Mdsds=-1.77512548973347*rou; 

Nu=0.00618430827275825*rou; Nv=1.31787983106965*rou; Nr=-2.12059813452114*rou;
Ndu=0.00432067452610559*rou; Ndv=2.54908610448936*rou; Ndr=-5.08662579871407*rou; 
Nvv=-0.599395502737668*rou;

 %刚体的质量惯性矩阵MRB
MRB=[m 0 0 0 m*zG -m*yG
     0 m 0 -m*zG 0 m*xG
     0 0 m m*yG -m*xG 0
     0 -m*zG m*yG Ix -Ixy -Ixz
     m*zG 0 -m*xG -Ixy Iy -Iyz
     -m*yG m*xG 0 -Ixz -Iyz Iz];   
%附加质量惯性矩阵
MA=-[Xdu Xdv Xdw 0 Xdq Xdr
           Ydu Ydv  0 0 0 Ydr
           Zdu 0 Zdw 0 Zdq 0
           0 Kdv Kdw Kdp 0 0
           Mdu 0 Mdw 0 Mdq 0
           Ndu Ndv 0 0 0 Ndr];        
Mv=MRB+MA;       

 %科里奥利力和向心力矩阵CRBv=Cv
 Cv=[0 0 0 m*(yG*q+zG*r) m*(w-xG*q) -m*(xG*r+v)
         0 0 0 -m*(w+yG*p) m*(zG*r+xG*p) m*(ux-yG*r)
         0 0 0 m*(v-zG*p) -m*(ux+zG*q) m*(xG*p+yG*q)
        -m*(yG*q+zG*r) m*(w+yG*p) m*(zG*p-v) 0 -Iyz*q-Ixz*p+Iz*r Iyz*r+Ixy*p-Iy*q
          m*(xG*q-w) -m*(zG*r+xG*p) m*(ux+zG*q) Iyz*q+Ixz*p-Iz*r 0 -Ixz*r-Ixy*q+Ix*p
          m*(xG*r+v) m*(yG*r-ux) -m*(xG*p+yG*q) -Iyz*r-Ixy*p+Iy*q Ixz*r+Ixy*q-Ix*p 0];
      
%粘滞阻力
Dv=-[Xu+Xuw*abs(w), Xv+Xvv*abs(v), Xw+Xds*(ds-pi/2*sign(ds))*abs(w), 0, Xq, Xr;
         Yu, Yv+Yvv*abs(v), 0, 0, 0, Yr;
         Zu, 0, Zw+Zww*abs(w)+Zdsds*(ds-pi/2*sign(ds))^2*abs(w), 0, Zq, 0;
         Kuw*abs(w), Kv, Kw, Kp, 0, 0;
         Mu+Muw*w, 0, Mw+Mww*abs(w)+Mdsds*(ds-pi/2*sign(ds))^2*abs(w)+Mds*(ds-pi/2*sign(ds))*w, 0, Mq, 0;
         Nu, Nv+Nvv*abs(v), 0, 0, 0, Nr];

%载体的恢复力/力矩
gv=[(W-B)*sin(th)
    -(W-B)*cos(th)*sin(fa)
    -(W-B)*cos(th)*cos(fa) 
    -(yG*W-yB*B)*cos(th)*cos(fa)+(zG*W-zB*B)*cos(th)*sin(fa)
    (zG*W-zB*B)*sin(th)+(xG*W-xB*B)*cos(th)*cos(fa)
    -(xG*W-xB*B)*cos(th)*sin(fa)-(yG*W-yB*B)*sin(th)];

%雅可比矩阵

JT=[cos(psi)*cos(th),sin(psi)*cos(th),-sin(th),0,0,0;
          cos(psi)*sin(th)*sin(fa)-sin(psi)*cos(fa), cos(psi)*cos(fa)+sin(fa)*sin(th)*sin(psi),cos(th)*sin(fa),0,0,0;
          sin(psi)*sin(fa)+cos(psi)*cos(fa)*sin(th), sin(th)*sin(psi)*cos(fa)-cos(psi)*sin(fa),cos(th)*cos(fa),0,0,0;
          0,0,0,1,0,0;
          0,0,0,sin(fa)*tan(th),cos(fa),sin(fa)/cos(th);
          0,0,0,cos(fa)*tan(th), -sin(fa),cos(fa)/cos(th)]; 
invJ=[cos(psi)*cos(th),sin(psi)*cos(th),-sin(th),0,0,0;
          cos(psi)*sin(th)*sin(fa)-sin(psi)*cos(fa), cos(psi)*cos(fa)+sin(fa)*sin(th)*sin(psi),cos(th)*sin(fa),0,0,0;
          sin(psi)*sin(fa)+cos(psi)*cos(fa)*sin(th), sin(th)*sin(psi)*cos(fa)-cos(psi)*sin(fa),cos(th)*cos(fa),0,0,0;
          0,0,0,1,0,-sin(th);
          0,0,0,0,cos(fa),sin(fa)*cos(th);
          0,0,0,0,-sin(fa),cos(fa)*cos(th)]; 
invJT=[cos(psi)*cos(th), cos(psi)*sin(th)*sin(fa)-sin(psi)*cos(fa), sin(psi)*sin(fa)+cos(psi)*cos(fa)*sin(th),0,0,0;
            sin(psi)*cos(th), cos(psi)*cos(fa)+sin(fa)*sin(th)*sin(psi),sin(th)*sin(psi)*cos(fa)-cos(psi)*sin(fa),0,0,0;
           -sin(th), cos(th)*sin(fa), cos(th)*cos(fa),0,0,0;
           0,0,0,1,0,0;
           0,0,0,0,cos(fa),-sin(fa);
           0,0,0,-sin(th),sin(fa)*cos(th),cos(fa)*cos(th)]; 
       
 %雅可比矩阵的导数，不清楚正不正确

dJ1=[0,sin(psi)*sin(fa)+cos(psi)*sin(th)*cos(fa),sin(psi)*cos(fa)-cos(psi)*sin(fa)*sin(th),0,0,0;
         0,-cos(psi)*sin(fa)+cos(fa)*sin(th)*sin(psi),-cos(psi)*cos(fa)-sin(th)*sin(psi)*sin(fa),0,0,0;
         0,cos(th)*cos(fa),-cos(th)*sin(fa),0,0,0;
         0,0,0,0,cos(fa)*tan(th),-sin(fa)*tan(th);
         0,0,0,0,-sin(fa),-cos(fa);
         0,0,0,0,cos(fa)/cos(th),-sin(fa)/cos(th)];  

dJ2=[-cos(psi)*sin(th),cos(psi)*cos(th)*sin(fa),cos(psi)*cos(fa)*cos(th),0,0,0;
          -sin(psi)*sin(th),sin(fa)*cos(th)*sin(psi),cos(th)*sin(psi)*cos(fa),0,0,0;
          -cos(th),-sin(th)*sin(fa),-sin(th)*cos(fa),0,0,0;
            0,0,0,0,sin(fa)*sec(th)^2,cos(fa)*sec(th)^2;
            0,0,0,0,0,0;
            0,0,0,0,sin(fa)*sec(th)*tan(th),cos(fa)*sec(th)*tan(th) ];

dJ3=[-sin(psi)*cos(th),-cos(psi)*cos(fa)-sin(psi)*sin(th)*sin(fa),cos(psi)*sin(fa)-sin(psi)*cos(fa)*sin(th),0,0,0;
          cos(psi)*cos(th),-sin(psi)*cos(fa)+sin(fa)*sin(th)*cos(psi),sin(psi)*sin(fa)+sin(th)*cos(psi)*cos(fa),0,0,0;    
          0,0,0,0,0,0;
          0,0,0,0,0,0;
          0,0,0,0,0,0;
          0,0,0,0,0,0];
dJ=dfa*dJ1+dth*dJ2+dpsi*dJ3;  

% Mv=diag([4108  14989  5821 1356  6020  8931]);

% Mv=[4108   -52        -64      0      -184     -67
%     120     2000    0        14      0        -1471
%     30        0          5821   -8      1279     0
%     0        -35       -38      1356   0         -38
%     48        0        -367      0       6020     0
%     3        -2692    0        -38      0          8931];

%名义值：运动坐标系转换到惯性坐标系下
% M=0.7*invJT*Mv*invJ;
C=(1+0.4)*invJT*(Cv-Mv*invJ*dJ)*invJ;
D=(1-0.4)*invJT*Dv*invJ;
g=(1-0.3)*invJT*gv;
mdisn=0.6*invJT*mdis_c;


%估算的S值
fx=C*deta+D*deta+g-mdisn;

end

== matlab function semi_GSTA/MATLAB Function7 ==
  data: Tv0 output; Tv input; t input
function Tv0= Tv_initial(Tv,t)

if t<0.5
    Tv0=Tv;
else
    Tv0=zeros(6,1);
end

end

== matlab function semi_GSTA/Subsystem3/TD4/fe ==
  data: x1 input; u output; x2 input; r input; h input
function u=fhan(x1,x2,r,h)
%eml
d=r*h*h;
a0=h*x2;
y=x1+a0;
a1=(d*(d+8*abs(y)))^0.5;
a2=a0+sign(y)*(a1-d)*0.5;
a=(a0+y)*(sign(y+d)-sign(y-d))*0.5+a2*(1-(sign(y+d)-sign(y-d))*0.5);
u=-r*(a/d)*(sign(a+d)-sign(a-d))*0.5-r*sign(a)*(1-(sign(a+d)-sign(a-d))*0.5);

== matlab function semi_GSTA/Subsystem3/TD5/fe ==
  data: x1 input; u output; x2 input; r input; h input
function u=fhan(x1,x2,r,h)
%eml
d=r*h*h;
a0=h*x2;
y=x1+a0;
a1=(d*(d+8*abs(y)))^0.5;
a2=a0+sign(y)*(a1-d)*0.5;
a=(a0+y)*(sign(y+d)-sign(y-d))*0.5+a2*(1-(sign(y+d)-sign(y-d))*0.5);
u=-r*(a/d)*(sign(a+d)-sign(a-d))*0.5-r*sign(a)*(1-(sign(a+d)-sign(a-d))*0.5);

== matlab function semi_GSTA/Subsystem3/TD6/fe ==
  data: x1 input; u output; x2 input; r input; h input
function u=fhan(x1,x2,r,h)
%eml
d=r*h*h;
a0=h*x2;
y=x1+a0;
a1=(d*(d+8*abs(y)))^0.5;
a2=a0+sign(y)*(a1-d)*0.5;
a=(a0+y)*(sign(y+d)-sign(y-d))*0.5+a2*(1-(sign(y+d)-sign(y-d))*0.5);
u=-r*(a/d)*(sign(a+d)-sign(a-d))*0.5-r*sign(a)*(1-(sign(a+d)-sign(a-d))*0.5);

== matlab function semi_GSTA/MATLAB Function15 ==
  data: usta input; detad input; ddetad input; eta input; deta input; Tv output; Tn output; fx input; c input; Mn input
function [Tv,Tn] = AGSTA(usta,detad,ddetad,eta,deta,fx,c,Mn)

fa=eta(4); th=eta(5); psi=eta(6);
de=deta-detad;

%旋转矩阵，惯性系下输入到体坐标系下转换
JT=[cos(psi)*cos(th),sin(psi)*cos(th),-sin(th),0,0,0;
          cos(psi)*sin(th)*sin(fa)-sin(psi)*cos(fa), cos(psi)*cos(fa)+sin(fa)*sin(th)*sin(psi),cos(th)*sin(fa),0,0,0;
          sin(psi)*sin(fa)+cos(psi)*cos(fa)*sin(th), sin(th)*sin(psi)*cos(fa)-cos(psi)*sin(fa),cos(th)*cos(fa),0,0,0;
          0,0,0,1,0,0;
          0,0,0,sin(fa)*tan(th),cos(fa),sin(fa)/cos(th);
          0,0,0,cos(fa)*tan(th), -sin(fa),cos(fa)/cos(th)]; 

cm=diag(c);
    
Tn=Mn*(ddetad-cm*de+usta)+fx;

%惯性下的输入转换到运动坐标系下的输入
Tv=JT*Tn;

end

== matlab function semi_GSTA/MATLAB Function14 ==
  data: k1 input; k2 input; x_k input; mu1 input; mu2 input; h input; v_k input; u_gsta output; u1_k output; u2_k output; q_sum output; q_multi output; v_kp1 output
function [u_gsta, u1_k, u2_k, q_sum, q_multi, v_kp1] = GSTA(k1, k2, x_k, mu1, mu2, h, v_k)


if  abs(x_k)==0
    q_sum = 0;
    q_multi = 0;
else
    lam_sum = - k1 * (mu1 * abs(x_k) ^ - 0.5 + mu2);                                                        
    lam_multi = k2 * (0.5 * mu1 * abs(x_k) ^ - 1 + 1.5 * mu1 * mu2 * abs(x_k) ^ - 0.5 + mu2^2 );
        
    q_sum = (2 - h * lam_sum ) / (1 - h * lam_sum + h ^ 2 * lam_multi ); 
    q_multi = 1 / (1 - h * lam_sum + h ^ 2 * lam_multi );
end

u1_k = q_sum - 1;    % u1_k=q1+q2-1;
u2_k = 1 / h * (u1_k - q_multi);   % u2_k=1/h*(u1_k-q1*q2);

v_kp1 = v_k + u2_k * x_k;
u_gsta = 1 / h * ( - x_k + u1_k * x_k ) + v_kp1;

end

== matlab function semi_GSTA/MATLAB Function20 ==
  data: eta input; deta output; v input
function deta = Kinematic(eta,v)

fa=eta(4); th=eta(5); psi=eta(6);

J=[cos(psi)*cos(th), cos(psi)*sin(th)*sin(fa)-sin(psi)*cos(fa), sin(psi)*sin(fa)+cos(psi)*cos(fa)*sin(th),0,0,0;
   sin(psi)*cos(th), cos(psi)*cos(fa)+sin(fa)*sin(th)*sin(psi),sin(th)*sin(psi)*cos(fa)-cos(psi)*sin(fa),0,0,0;
   -sin(th), cos(th)*sin(fa), cos(th)*cos(fa),0,0,0;
   0,0,0,1,sin(fa)*tan(th),cos(fa)*tan(th);
   0,0,0,0,cos(fa),-sin(fa);
   0,0,0,0,sin(fa)*sec(th),cos(fa)*sec(th)];  

deta=J*v;

end

== matlab function semi_GSTA/MATLAB Function31 ==
  data: chattering output; Tv_kp1 input; Tv_k1 input; chattering_last input
function chattering= variation(Tv_kp1,Tv_k1,chattering_last)

variation_c_kp1 =abs(Tv_kp1-Tv_k1);
chattering=variation_c_kp1+chattering_last;
end
